simulink model "UAV_Dynamics"  (R2023b)
settings: Solver=ode4  StartTime=0.0  StopTime=inf  RelTol=1e-3
model workspace (MAT data in the model file):
  Horizontal_position_accuracy = 0.01
  Horizontal_position_accuracy_fault = Simulink.Parameter
  Horizontal_position_accuracy_fault.Value = 0
  Horizontal_position_accuracy_fault.DataType = 'auto'
  Horizontal_position_accuracy_fault.Complexity = 'real'
  Horizontal_position_accuracy_fault.Dimensions = [1 1]
  Velocity_accuracy = 0.01
  Velocity_accuracy_fault = Simulink.Parameter
  Velocity_accuracy_fault.Value = 0
  Velocity_accuracy_fault.DataType = 'auto'
  Velocity_accuracy_fault.Complexity = 'real'
  Velocity_accuracy_fault.Dimensions = [1 1]
  Vertical_position_accuracy = 0.01
  Vertical_position_accuracy_fault = Simulink.Parameter
  Vertical_position_accuracy_fault.Value = 0
  Vertical_position_accuracy_fault.DataType = 'auto'
  Vertical_position_accuracy_fault.Complexity = 'real'
  Vertical_position_accuracy_fault.Dimensions = [1 1]
  bias_acc = [0 0 0]
  bias_gyro = [0 0 0]
  mag_bias = [0 0 0]
undefined symbols (not defined in the file): contact, control, ddx, ddy, ddz, dragCoeffMov, dx, dy, dz, fractalcoef, g, m_to_mm, mass, p, pitch, q, r, ref_height, ref_lat, ref_lon, roll, rotorDir, rotorPositions, rotorThrustMax, rotorTimeConst, rotorTorqueMax, SampleTime, windVel, X, Y, yaw, Z
libraries: aerolibatmos2 x1, sensorgpslib x1, robotcorelib x1, mspsensorlib x1, shared6dof x1, simulink x1
(part 1 of 2)
settings Model: Creator=The MathWorks, Inc.  LastModifiedBy=cardo
settings SolverCC: ZeroCrossControl=EnableAll  MaxZcPerStep=1
settings OptimizationCC: ReuseModelBlockBuffer=off
settings ModelReferenceCC: EnableRefExpFcnMdlSchedulingChecks=on
settings RTWCC: DLArmComputeVersion=19.05

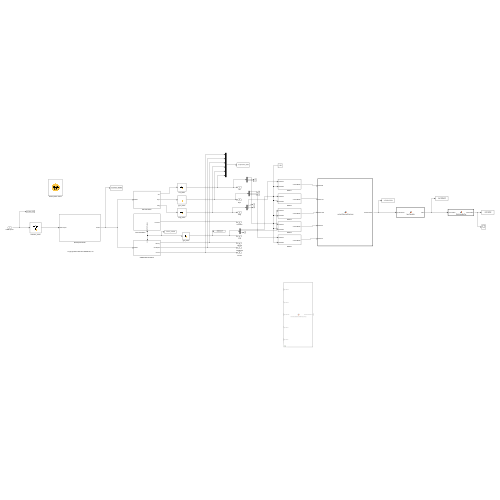
[thumbnail: Simulink's stored preview of the top-level diagram]
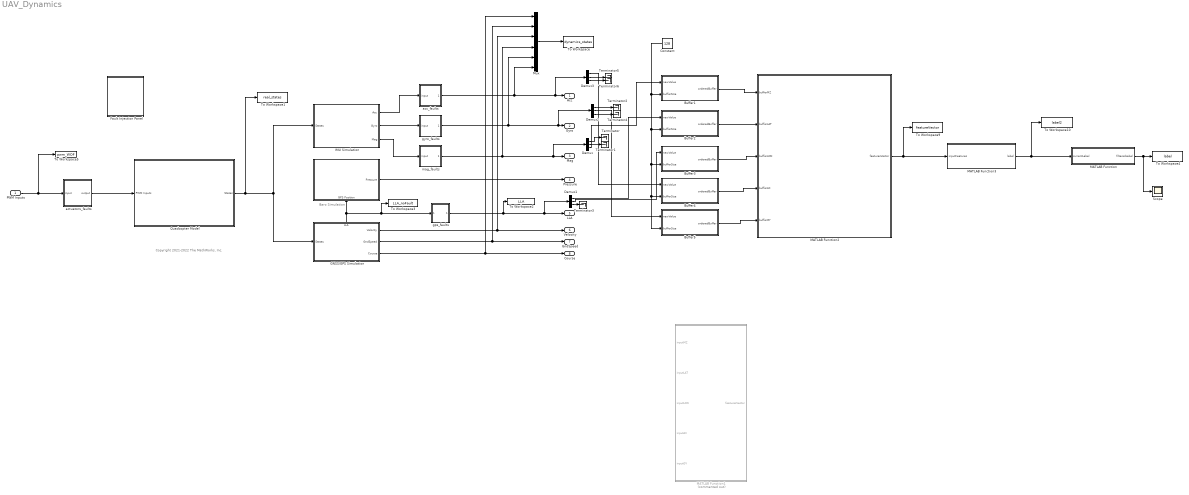
== system UAV_Dynamics ==
  note: Baro Simulation
  note: Copyright 2021-2022 The MathWorks, Inc.
  PWM Inputs : Inport
  " " : Subsystem
      settings: PortSchema="{\"entries\":[{\"content\":{\"sides\":[{\"content\":{\"connectorIds\":[]},\"type\":\"ConnectorPlacement.EquallySpacedRectSide\",\"uuid\":\"7ecc8b21-8f8f-4144-826a-6b68e30dbf7d\"},{\"content\":{\"connectorIds\":[\"Out1\"],\"side\":\"RIGHT\"},\"type\":\"ConnectorPlacement.EquallySpacedRectSide\",\"uuid\":\"81a1dd55-8330-4386-9921-36c0eb60d526\"},{\"content\":{\"connectorIds\":[],\"side\":\"TOP\"},\"type\":\"ConnectorPlacement.EquallySpacedRectSide\",\"uuid\":\"b99caff5-b40d-407d-b30e-35210c1aee1d\"},{\"content\":{\"connectorIds\":[\"In1\"],\"side\":\"BOTTOM\"},\"type\":\"ConnectorPlacement.EquallySpacedRectSide\",\"uuid\":\"18bfda3d-4fab-4e61-9ebc-e384e51de306\"}]},\"type\":\"ConnectorPlacement.EquallySpacedConnector\",\"uuid\":\"17ab4e96-b761-4c62-a0bb-ab626dac3eaa\"}],\"packageUris\":[\"http://schema.mathworks.com/mf0/Connector/R2020b\"],\"version\":\"1.0\"}"
  Buffer1 : Subsystem
  Buffer2 : Subsystem
  Buffer3 : Subsystem
  Buffer4 : Subsystem
  Buffer5 : Subsystem
  Constant : Constant  Value=128  SampleTime=0.01
  Demux{,1..3} (4 alike) : Demux  Outputs=3
  Fault Injection Panel : Subsystem
      mask DialogControl Container3 Prompt: Fault Injection
      mask DialogControl Control3 Prompt: Fault Injection Actuators
      mask DialogControl Control4 Prompt: Faut Injection Actuators
      mask DialogControl Control4 Callback: open_system('UAV_Dynamics/actuators_faults', 'mask');
      mask DialogControl Control5 Prompt: Fault Injection Sensors
      mask DialogControl Control6 Prompt: Fault Injection Accelometer
      mask DialogControl Control6 Callback: open_system('UAV_Dynamics/acc_faults', 'mask');
      mask DialogControl Control7 Prompt: Fault Injection Gyroscope
      mask DialogControl Control7 Callback: open_system('UAV_Dynamics/gyro_faults', 'mask');
      mask DialogControl Control8 Prompt: Fault Injection Magnometer
      mask DialogControl Control8 Callback: open_system('UAV_Dynamics/mag_faults', 'mask');
      mask DialogControl Control9 Prompt: Fault Injection GPS
      mask DialogControl Control9 Callback: open_system('UAV_Dynamics/gps_faults', 'mask');
  GNSS/GPS Simulation : Subsystem
      settings: PortSchema="{\"entries\":[{\"content\":{\"sides\":[{\"content\":{\"connectorIds\":[\"In1\"]},\"type\":\"ConnectorPlacement.EquallySpacedRectSide\",\"uuid\":\"4934e8ff-5d4b-4e11-968d-c23bd62383a0\"},{\"content\":{\"connectorIds\":[\"Out1\",\"Out2\",\"Out3\"],\"side\":\"RIGHT\"},\"type\":\"ConnectorPlacement.EquallySpacedRectSide\",\"uuid\":\"9ec8bc0a-2d3c-4dca-835c-010ac29b6ebc\"},{\"content\":{\"connectorIds\":[\"Out4\"],\"side\":\"TOP\"},\"type\":\"ConnectorPlacement.EquallySpacedRectSide\",\"uuid\":\"04f09eb4-1bd9-450e-b951-47054bdd92ad\"}]},\"type\":\"ConnectorPlacement.EquallySpacedConnector\",\"uuid\":\"9a5920cf-a58d-4c98-839b-fbac94edbe7e\"}],\"packageUris\":[\"http://schema.mathworks.com/mf0/Connector/R2020b\"],\"version\":\"1.0\"}"
  IMU Simulation : Subsystem
  MATLAB Function : MATLAB Function  TreatAsAtomicUnit=on
  MATLAB Function1 : MATLAB Function  Commented=on  TreatAsAtomicUnit=on
  MATLAB Function2 : MATLAB Function  TreatAsAtomicUnit=on
  MATLAB Function3 : MATLAB Function  TreatAsAtomicUnit=on
  Mux : Mux  Inputs=6
  Quadcopter Model : Subsystem
  Scope : Scope
  Terminator{,1..6} (7 alike) : Terminator
  To Workspace : ToWorkspace  VariableName=dynamics_states  SaveFormat=Timeseries  SampleTime=0.01
  To Workspace1 : ToWorkspace  VariableName=real_states  SaveFormat=Timeseries  SampleTime=0.01
  To Workspace10 : ToWorkspace  VariableName=label2  SaveFormat=Timeseries  SampleTime=-1
  To Workspace2 : ToWorkspace  VariableName=LLA  SaveFormat=Timeseries  SampleTime=0.01
  To Workspace3 : ToWorkspace  VariableName=LLA_noFault  SaveFormat=Timeseries  SampleTime=0.01
  To Workspace4 : ToWorkspace  VariableName=label  SaveFormat=Timeseries  SampleTime=-1
  To Workspace5 : ToWorkspace  VariableName=pwm_WOF  SaveFormat=Timeseries  SampleTime=0.01
  To Workspace9 : ToWorkspace  VariableName=featureVector  SaveFormat=Timeseries  SampleTime=-1
  acc_faults : Subsystem  mask{tf=100, freezingX=off, freezingY=off, freezingZ=off, accuracyX=off, accuracyY=off, accuracyZ=off, d_accuracy=10.0, driftX=off, driftY=off, driftZ=off, landa=0.07, biasX=off, bias_ax=0, biasY=off, bias_ay=0.01, biasZ=off, bias_az=0}
      mask prompts: tf "Fault Time(s):"; freezingX "Freezing Fault ax On"; freezingY "Freezing Fault ay On"; freezingZ "Freezing Fault az On"; accuracyX "Accuracy Fault ax On"; accuracyY "Accuracy Fault ay On"; accuracyZ "Accuracy Fault az On"; d_accuracy "Accuracy Error max, dmax (%):"; driftX "Drift Fault ax On"; driftY "Drift Fault ay On"; driftZ "Drift Fault az On"; landa "Lambda:"; biasX "Bias Fault ax On"; bias_ax "Bias Offset ax (m/s²):"; biasY "Bias Fault ay On"; bias_ay "Bias Offset ay (m/s²):"; biasZ "Bias Fault az On"; bias_az "Bias Offset az (m/s²):"
      mask TypeOptions tf: tf/Value
      mask DialogControl Control5 Prompt: Fault Injection Accelerometer
      mask DialogControl Container7 Prompt: Fault Time
      mask DialogControl Control4 Prompt: Insert the Fault Time
      mask DialogControl ParameterGroupVar Prompt: Fault Type
      mask DialogControl DescTextVar Prompt: Select the type of Fault,its amplitude and the relative axis
      mask DialogControl Container4 Prompt: Freezing Fault
      mask DialogControl Control6_copy_copy Prompt: Insert Freezing Fault
      mask DialogControl Container5 Prompt: Accuracy Fault
      mask DialogControl Control6_copy_copy_copy Prompt: Insert Accuracy Fault. Select the axis with the Fault and write the percent of max error
      mask DialogControl Control3 Prompt: y(t) = x(t) + d(t), |d(t)| ≤ dmax, for all t ≥ tf
      mask DialogControl Container6 Prompt: Drift Fault
      mask DialogControl Control6_copy Prompt: Insert Drift Offset Fault. Select the axis with the Fault and write the value of lambda.
      mask DialogControl Control2 Prompt: y(t) = x(t) + d(t), |d(t)| = λ*t, 0 < λ << 1, for all t ≥ tf
      mask DialogControl Container8 Prompt: Bias Fault
      mask DialogControl Control6 Prompt: Insert Bias Offset Fault
      mask Display: image('accelometer_fault_icon.png');
  actuators_faults : Subsystem  mask{tf=150, num_motor=No Fault, lock_in_place=off, float=off, handover=off, loss_effectiveness=off, perc=30}
      mask prompts: tf "Fault Time(s):"; lock_in_place "Lock in Place Fault On"; float "Float Fault On"; handover "Handover Fault On"; loss_effectiveness "Loss of Effectiveness Fault On"; perc "Percentage of Fault (%):"
      mask TypeOptions tf: tf/Value
      mask DialogControl DescTextVar Prompt: Actuators Fault Injection
      mask DialogControl ParameterGroupVar Prompt: Fault Time and Motor
      mask DialogControl Control2 Prompt: Insert the fault time
      mask DialogControl Control3 Prompt: Insert the actuator with the fault
      mask DialogControl Container3 Prompt: Fault Type
      mask DialogControl Container5 Prompt: Lock in Place
      mask DialogControl Container6 Prompt: Float
      mask DialogControl Container7 Prompt: Handover
      mask DialogControl Container8 Prompt: Loss of Effectiveness
      mask Display: image('motor_fault.png');
  gps_faults : Subsystem  mask{tf=100, loss_signal=off, lossProbability=20, gps_accuracy=on, AccuracyErrorMeters=5}
      mask prompts: tf "Fault Time (s):"; loss_signal "Packet Loss Signal On"; lossProbability "Probability of Packet Loss of Signal"; gps_accuracy "GPS Fault On"; AccuracyErrorMeters "Error Position accuracy (m):"
      mask TypeOptions tf: tf/Value
      mask DialogControl Control5 Prompt: Fault Injection GPS
      mask DialogControl Container7 Prompt: Fault Time
      mask DialogControl Control4 Prompt: Insert the fault time
      mask DialogControl ParameterGroupVar Prompt: Fault
      mask DialogControl DescTextVar Prompt: Select the Fault Type and its amplitude
      mask DialogControl Container8 Prompt: Packet Loss of Signal
      mask DialogControl Container5 Prompt: GPS Accuracy
      mask Display: image('gps_fault_icon.png');
  gyro_faults : Subsystem  mask{tf=100, freezingX=off, freezingY=off, freezingZ=off, accuracyX=off, accuracyY=off, accuracyZ=off, d_accuracy=10.0, driftX=off, driftY=off, driftZ=off, landa=0.01, biasX=off, bias_gx=0, biasY=off, bias_gy=0.06, biasZ=off, bias_gz=0}
      mask prompts: tf "Fault Time (s):"; freezingX "Freezing Fault gx On"; freezingY "Freezing Fault gy On"; freezingZ "Freezing Fault gz On"; accuracyX "Accuracy Fault gx On"; accuracyY "Accuracy Fault gy On"; accuracyZ "Accuracy Fault gz On"; d_accuracy "Accuracy Error max, dmax (%):"; driftX "Drift Fault gx On"; driftY "Drift Fault gy On"; driftZ "Drift Fault gz On"; landa "Lambda"; biasX "Bias Fault gx On"; bias_gx "Bias Offset gx (rad/s):"; biasY "Bias Fault gy On"; bias_gy "Bias Offset gy (rad/s):"; biasZ "Bias Fault gz On"; bias_gz "Bias Offset gz (rad/s):"
      mask TypeOptions tf: tf/Value
      mask DialogControl Control5 Prompt: Fault Injection Gyroscope
      mask DialogControl Container7 Prompt: Fault Time
      mask DialogControl Control4 Prompt: Insert the Fault Time
      mask DialogControl ParameterGroupVar Prompt: Fault Type
      mask DialogControl DescTextVar Prompt: Select the type of Fault,its amplitude and the relative axis
      mask DialogControl Container4 Prompt: Freezing Fault
      mask DialogControl Control6_copy_copy Prompt: Insert Freezing Fault
      mask DialogControl Container5 Prompt: Accuracy Fault
      mask DialogControl Control6_copy_copy_copy Prompt: Insert Accuracy Fault. Select the axis with the Fault and write the percent of max error
      mask DialogControl Control3 Prompt: y(t) = x(t) + d(t), |d(t)| ≤ dmax, for all t ≥ tf
      mask DialogControl Container6 Prompt: Drift Fault
      mask DialogControl Control6_copy Prompt: Insert Drift Offset Fault. Select the axis with the Fault and write the value of lambda.
      mask DialogControl Control2 Prompt: y(t) = x(t) + d(t), |d(t)| = λ*t, 0 < λ << 1, for all t ≥ tf
      mask DialogControl Container8 Prompt: Bias Fault
      mask DialogControl Control6 Prompt: Insert Bias Offset Fault
      mask Display: image('gyroscope_fault_icon.png');
  mag_faults : Subsystem  mask{tf=100, freezingX=off, freezingY=off, freezingZ=off, accuracyX=off, accuracyY=off, accuracyZ=off, d_accuracy=20, driftX=off, driftY=off, driftZ=off, landa=0.1, biasX=off, bias_mx=0, biasY=off, bias_my=0, biasZ=off, bias_mz=0}
      mask prompts: tf "Fault Time (s):"; freezingX "Freezing Fault mx On"; freezingY "Freezing Fault my On"; freezingZ "Freezing Fault mz On"; accuracyX "Accuracy Fault mx On"; accuracyY "Accuracy Fault my On"; accuracyZ "Accuracy Fault mz On"; d_accuracy "Accuracy Error max, dmax (%):"; driftX "Drift Fault mx On"; driftY "Drift Fault my On"; driftZ "Drift Fault mz On"; landa "Lambda:"; biasX "Bias Fault mx On"; bias_mx "Bias Offset mx (µT):"; biasY "Bias Fault my On"; bias_my "Bias Offset my (µT):"; biasZ "Bias Fault mz On"; bias_mz "Bias Offset mz (µT):"
      mask TypeOptions tf: tf/Value
      mask DialogControl Control5 Prompt: Fault Injection Magnometer
      mask DialogControl Container7 Prompt: Fault Time
      mask DialogControl Control4 Prompt: Insert the Fault Time
      mask DialogControl ParameterGroupVar Prompt: Fault Type
      mask DialogControl DescTextVar Prompt: Select the type of Fault,its amplitude and the relative axis
      mask DialogControl Container4 Prompt: Freezing Fault
      mask DialogControl Control6_copy_copy Prompt: Insert Freezing Fault
      mask DialogControl Container5 Prompt: Accuracy Fault
      mask DialogControl Control6_copy_copy_copy Prompt: Insert Accuracy Fault. Select the axis with the Fault and write the percent of max error
      mask DialogControl Control3 Prompt: y(t) = x(t) + d(t), |d(t)| ≤ dmax, for all t ≥ tf
      mask DialogControl Container6 Prompt: Drift Fault
      mask DialogControl Control6_copy Prompt: Insert Drift Offset Fault. Select the axis with the Fault and write the value of lambda.
      mask DialogControl Control2 Prompt: y(t) = x(t) + d(t), |d(t)| = λ*t, 0 < λ << 1, for all t ≥ tf
      mask DialogControl Container8 Prompt: Bias Fault
      mask DialogControl Control6 Prompt: Insert Bias Offset Fault
      mask Display: image('magnometer_fault_icon.png');
  Acc : Outport
  Gyro : Outport  Port=2
  Mag : Outport  Port=3
  Pressure : Outport  Port=4
  LLA : Outport  Port=5
  Velocity : Outport  Port=6
  GndSpeed : Outport  Port=7
  Course : Outport  Port=8
  wires:
  IMU Simulation/2(Gyro) -> gyro_faults/1(input)
  IMU Simulation/3(Mag) -> mag_faults/1(input)
  " "/1(Pressure) -> Pressure/1
  GNSS/GPS Simulation/1(Velocity) -> Mux/3, Velocity/1
  GNSS/GPS Simulation/2(GndSpeed) -> Mux/2, GndSpeed/1
  GNSS/GPS Simulation/3(Course) -> Mux/1, Course/1
  Mux/1 -> To Workspace/1
  IMU Simulation/1(Acc) -> acc_faults/1(input)
  actuators_faults/1(output) -> Quadcopter Model/1(PWM Inputs)
  mag_faults/1(output) -> Mux/4, Demux/1, Mag/1
  GNSS/GPS Simulation/4(LLA) -> gps_faults/1(input), To Workspace3/1, " "/1(GPS Position)
  Quadcopter Model/1(States) -> To Workspace1/1, GNSS/GPS Simulation/1(States), IMU Simulation/1(States)
  Demux/1 -> Terminator/1
  Demux/2 -> Terminator1/1
  PWM Inputs/1 -> To Workspace5/1, actuators_faults/1(input)
  Demux2/3 -> Terminator4/1
  gyro_faults/1(output) -> Mux/5, Demux2/1, Gyro/1
  Demux2/1 -> Terminator2/1
  acc_faults/1(output) -> Mux/6, Demux3/1, Acc/1
  Demux3/3 -> Terminator6/1
  gps_faults/1(output) -> Demux1/1, LLA/1, To Workspace2/1
  Demux1/3 -> Terminator3/1
  Demux3/2 -> Terminator5/1
  MATLAB Function3/1(label) -> MATLAB Function/1(currentLabel), To Workspace10/1
  Buffer4/1(orderedBuffer) -> MATLAB Function2/4(bufferAX)
  Buffer5/1(orderedBuffer) -> MATLAB Function2/5(bufferGY)
  Buffer3/1(orderedBuffer) -> MATLAB Function2/3(bufferLON)
  Buffer1/1(orderedBuffer) -> MATLAB Function2/1(bufferMZ)
  Buffer2/1(orderedBuffer) -> MATLAB Function2/2(bufferLAT)
  Constant/1 -> Buffer1/2(bufferSize), Buffer2/2(bufferSize), Buffer3/2(bufferSize), Buffer4/2(bufferSize), Buffer5/2(bufferSize)
  Demux/3 -> Buffer1/1(newValue)
  Demux1/1 -> Buffer2/1(newValue)
  Demux1/2 -> Buffer3/1(newValue)
  Demux3/1 -> Buffer4/1(newValue)
  Demux2/2 -> Buffer5/1(newValue)
  MATLAB Function2/1(featuresVector) -> MATLAB Function3/1(inputFeatures), To Workspace9/1
  MATLAB Function/1(filteredLabel) -> Scope/1, To Workspace4/1

== system UAV_Dynamics/  ==
  GPS Position : Inport
  Extract Altitude : Selector  InputPortWidth=3  IndexOptions=Index vector (dialog)  Indices=[3]  OutputSizes=1
  Gain1 : Gain  Gain=1/m_to_mm
  Gain2 : Gain  Gain=m_to_mm
  Lapse Rate Model : aerolibatmos2/ISA Atmosphere Model  useExtended=off  action=Warning  custom=on  viscosityOut=off  g=9.80665  gamma=1.4  R=287.0531  L=0.0065  h_trop=11000  h_strat=20000  rho0=1.225  P0=101325  T0=288.15  h0=0
  Random Number1 : RandomNumber  Variance=10000  Seed=10  SampleTime=SampleTime
  Sum1 : Sum  Inputs=|++
  Terminator : Terminator
  Terminator1 : Terminator
  Terminator2 : Terminator
  Pressure : Outport
  wires:
  Lapse Rate Model/2 -> Terminator1/1
  Lapse Rate Model/4 -> Terminator2/1
  Lapse Rate Model/1 -> Terminator/1
  Lapse Rate Model/3 -> Pressure/1
  Sum1/1 -> Gain1/1
  Gain2/1 -> Sum1/1
  Extract Altitude/1 -> Gain2/1
  Gain1/1 -> Lapse Rate Model/1
  GPS Position/1 -> Extract Altitude/1
  Random Number1/1 -> Sum1/2  "Pressure_noise"

== system UAV_Dynamics/Buffer1 ==
  newValue : Inport
  bufferSize : Inport  Port=2
  Delay : Delay  DelayLength=1  InitialCondition=1
  Delay1 : Delay  DelayLength=1  InitialCondition=zeros(128,1)
  MATLAB Function : MATLAB Function  TreatAsAtomicUnit=on
  MATLAB Function2 : MATLAB Function  TreatAsAtomicUnit=on
  orderedBuffer : Outport
  wires:
  newValue/1 -> MATLAB Function/2(newValue)
  MATLAB Function/1(buffer) -> Delay1/1, MATLAB Function2/1(buffer)
  MATLAB Function2/1(orderedBuffer) -> orderedBuffer/1
  MATLAB Function/2(k) -> Delay/1, MATLAB Function2/2(k)
  Delay/1 -> MATLAB Function/4("k ")
  Delay1/1 -> MATLAB Function/1("buffer ")
  bufferSize/1 -> MATLAB Function/3(bufferSize)

== system UAV_Dynamics/Buffer2 ==
  newValue : Inport
  bufferSize : Inport  Port=2
  Delay : Delay  DelayLength=1  InitialCondition=1
  Delay1 : Delay  DelayLength=1  InitialCondition=zeros(128,1)
  MATLAB Function : MATLAB Function  TreatAsAtomicUnit=on
  MATLAB Function2 : MATLAB Function  TreatAsAtomicUnit=on
  orderedBuffer : Outport
  wires:
  newValue/1 -> MATLAB Function/2(newValue)
  MATLAB Function/1(buffer) -> Delay1/1, MATLAB Function2/1(buffer)
  MATLAB Function2/1(orderedBuffer) -> orderedBuffer/1
  MATLAB Function/2(k) -> Delay/1, MATLAB Function2/2(k)
  Delay/1 -> MATLAB Function/4("k ")
  Delay1/1 -> MATLAB Function/1("buffer ")
  bufferSize/1 -> MATLAB Function/3(bufferSize)

== system UAV_Dynamics/Buffer3 ==
  newValue : Inport
  bufferSize : Inport  Port=2
  Delay : Delay  DelayLength=1  InitialCondition=1
  Delay1 : Delay  DelayLength=1  InitialCondition=zeros(128,1)
  MATLAB Function : MATLAB Function  TreatAsAtomicUnit=on
  MATLAB Function2 : MATLAB Function  TreatAsAtomicUnit=on
  orderedBuffer : Outport
  wires:
  newValue/1 -> MATLAB Function/2(newValue)
  MATLAB Function/1(buffer) -> Delay1/1, MATLAB Function2/1(buffer)
  MATLAB Function2/1(orderedBuffer) -> orderedBuffer/1
  MATLAB Function/2(k) -> Delay/1, MATLAB Function2/2(k)
  Delay/1 -> MATLAB Function/4("k ")
  Delay1/1 -> MATLAB Function/1("buffer ")
  bufferSize/1 -> MATLAB Function/3(bufferSize)

== system UAV_Dynamics/Buffer4 ==
  newValue : Inport
  bufferSize : Inport  Port=2
  Delay : Delay  DelayLength=1  InitialCondition=1
  Delay1 : Delay  DelayLength=1  InitialCondition=zeros(128,1)
  MATLAB Function : MATLAB Function  TreatAsAtomicUnit=on
  MATLAB Function2 : MATLAB Function  TreatAsAtomicUnit=on
  orderedBuffer : Outport
  wires:
  newValue/1 -> MATLAB Function/2(newValue)
  MATLAB Function/1(buffer) -> Delay1/1, MATLAB Function2/1(buffer)
  MATLAB Function2/1(orderedBuffer) -> orderedBuffer/1
  MATLAB Function/2(k) -> Delay/1, MATLAB Function2/2(k)
  Delay/1 -> MATLAB Function/4("k ")
  Delay1/1 -> MATLAB Function/1("buffer ")
  bufferSize/1 -> MATLAB Function/3(bufferSize)

== system UAV_Dynamics/Buffer5 ==
  newValue : Inport
  bufferSize : Inport  Port=2
  Delay : Delay  DelayLength=1  InitialCondition=1
  Delay1 : Delay  DelayLength=1  InitialCondition=zeros(128,1)
  MATLAB Function : MATLAB Function  TreatAsAtomicUnit=on
  MATLAB Function2 : MATLAB Function  TreatAsAtomicUnit=on
  orderedBuffer : Outport
  wires:
  newValue/1 -> MATLAB Function/2(newValue)
  MATLAB Function/1(buffer) -> Delay1/1, MATLAB Function2/1(buffer)
  MATLAB Function2/1(orderedBuffer) -> orderedBuffer/1
  MATLAB Function/2(k) -> Delay/1, MATLAB Function2/2(k)
  Delay/1 -> MATLAB Function/4("k ")
  Delay1/1 -> MATLAB Function/1("buffer ")
  bufferSize/1 -> MATLAB Function/3(bufferSize)

== system UAV_Dynamics/Fault Injection Panel ==

== system UAV_Dynamics/GNSS//GPS Simulation ==
  States : Inport
  Bus Selector : BusSelector  OutputSignals=dx,dy,dz  OutputAsBus=on
  Bus Selector1 : BusSelector  OutputSignals=X,Y,Z  OutputAsBus=on
  GPS : sensorgpslib/GPS  DispRefFrame=NED  PositionInputFormat=Local  ReferenceLocation=[ref_lat ref_lon ref_height]  HorizontalPositionAccuracy=0.01  VerticalPositionAccuracy=0.01  VelocityAccuracy=0.01  DecayFactor=0.99  SeedDouble=67  SimulateUsing=Code generation
  Reshape1 : Reshape  OutputDimensionality=Row vector (2-D)
  Reshape3 : Reshape  OutputDimensionality=Row vector (2-D)
  Velocity : Outport
  GndSpeed : Outport  Port=2
  Course : Outport  Port=3
  LLA : Outport  Port=4
  wires:
  Reshape3/1 -> GPS/1
  GPS/1 -> LLA/1  "lla"
  Bus Selector1/1 -> Reshape3/1
  Bus Selector/1 -> Reshape1/1
  Reshape1/1 -> GPS/2
  GPS/2 -> Velocity/1
  States/1 -> Bus Selector/1, Bus Selector1/1
  GPS/3 -> GndSpeed/1
  GPS/4 -> Course/1

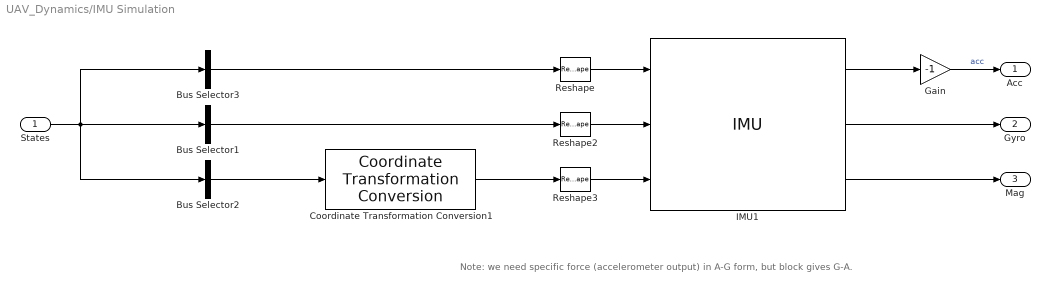
== system UAV_Dynamics/IMU Simulation ==
  note: Note:
      | we need specific force (accelerometer output) in A-G form, but block gives G-A.
  States : Inport
  Bus Selector1 : BusSelector  OutputSignals=p,q,r  OutputAsBus=on
  Bus Selector2 : BusSelector  OutputSignals=yaw,pitch,roll  OutputAsBus=on
  Bus Selector3 : BusSelector  OutputSignals=ddx,ddy,ddz  OutputAsBus=on
  Coordinate Transformation Conversion1 : robotcorelib/Coordinate Transformation Conversion  InputRepresentation=Euler Angles  InputEulerSequence=ZYX  ShowTrVecInputPort=on  OutputRepresentation=Quaternion  OutputEulerSequence=ZYX  ShowTrVecOutputPort=on  SimulateUsing=Interpreted execution
  Gain : Gain  Gain=-1
  IMU1 : mspsensorlib/IMU  DispRefFrame=NED  TemperaturePort=off  Temperature=25  MagneticFieldPort=off  MagneticFieldNED=[21.5 1.16 43.1]  MagneticFieldENU=[ -2.4169, 27.5550, 16.0849 ]  SeedDouble=87254  SimulateUsing=Interpreted execution  AccelParamsMeasurementRange=Inf  AccelParamsResolution=0  AccelParamsConstantBias=[ 0, 0, 0]  AccelParamsAxesMisalignment=[ 0, 0, 0 ]  AccelParamsNoiseDensity=0.0003  AccelParamsBiasInstability=[ 0, 0, 0 ]  AccelParamsBiasInstabilityNumerator=fractalcoef().Numerator  AccelParamsBiasInstabilityDenominator=fractalcoef().Denominator  AccelParamsRandomWalk=[ 0, 0, 0 ]  AccelParamsNoiseType=double-sided  AccelParamsTemperatureBias=[ 0, 0, 0 ]  AccelParamsTemperatureScaleFactor=[ 0, 0, 0 ]  GyroParamsMeasurementRange=Inf  GyroParamsResolution=0  GyroParamsConstantBias=[ 0, 0, 0]  GyroParamsAxesMisalignment=[ 0, 0, 0 ]  GyroParamsAccelerationBias=0.0001  GyroParamsNoiseDensity=0.01  GyroParamsBiasInstability=[ 0, 0, 0 ]  GyroParamsBiasInstabilityNumerator=fractalcoef().Numerator  GyroParamsBiasInstabilityDenominator=fractalcoef().Denominator  GyroParamsRandomWalk=[ 0, 0, 0 ]  GyroParamsNoiseType=double-sided  GyroParamsTemperatureBias=[ 0, 0, 0 ]  GyroParamsTemperatureScaleFactor=[ 0, 0, 0 ]  MagParamsMeasurementRange=Inf  MagParamsResolution=0  MagParamsConstantBias=[ 0, 0, 0]  MagParamsAxesMisalignment=[ 0, 0, 0 ]  MagParamsNoiseDensity=0.0005  MagParamsBiasInstability=[ 0, 0, 0 ]  MagParamsBiasInstabilityNumerator=fractalcoef().Numerator  MagParamsBiasInstabilityDenominator=fractalcoef().Denominator  MagParamsRandomWalk=[ 0, 0, 0 ]  MagParamsNoiseType=double-sided  MagParamsTemperatureBias=[ 0, 0, 0 ]  MagParamsTemperatureScaleFactor=[ 0, 0, 0 ]
  Reshape : Reshape  OutputDimensionality=Row vector (2-D)
  Reshape2 : Reshape  OutputDimensionality=Row vector (2-D)
  Reshape3 : Reshape  OutputDimensionality=Row vector (2-D)
  Acc : Outport
  Gyro : Outport  Port=2
  Mag : Outport  Port=3
  wires:
  Coordinate Transformation Conversion1/1 -> Reshape3/1
  Reshape3/1 -> IMU1/3
  IMU1/3 -> Mag/1
  IMU1/2 -> Gyro/1
  Reshape/1 -> IMU1/1
  Bus Selector3/1 -> Reshape/1
  IMU1/1 -> Gain/1
  Bus Selector1/1 -> Reshape2/1
  Bus Selector2/1 -> Coordinate Transformation Conversion1/1
  Reshape2/1 -> IMU1/2
  States/1 -> Bus Selector1/1, Bus Selector2/1, Bus Selector3/1
  Gain/1 -> Acc/1  "acc"

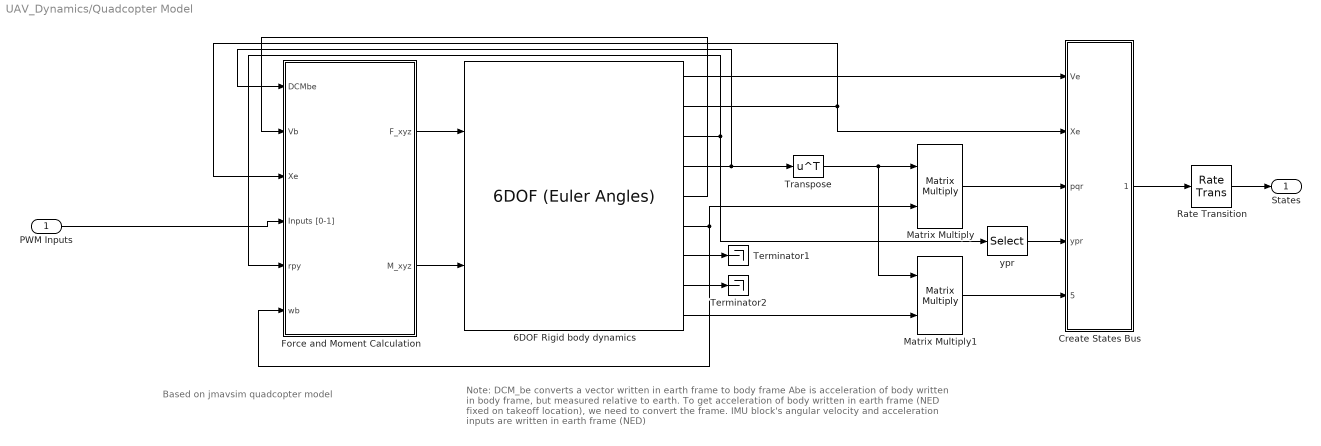
== system UAV_Dynamics/Quadcopter Model ==
  note: Note:
      | DCM_be converts a vector written in earth frame to body frame
      | Abe is acceleration of body written in body frame, but measured relative to earth.
      | To get acceleration of body written in earth frame (NED fixed on takeoff location), we need to convert the frame.
      | IMU block's angular velocity and acceleration inputs are written in earth frame (NED)
  note: Based on jmavsim quadcopter model
  PWM Inputs : Inport
  "6DOF Rigid body dynamics " : shared6dof/6DOF (Euler Angles)  units=Metric (MKS)  mtype=Fixed  rep=Quaternion  xme_0=init.posNED  Vm_0=init.vb  eul_0=init.euler  pm_0=init.angRates  mass_0=mass  mass_e=0.5  mass_f=2.0  inertia=inertia  inertia_e=eye(3)  inertia_f=2*eye(3)  k_quat=1  vre_flag=on  abi_flag=on  aMode=aMode  xme_statename=''  Vm_statename=''  eul_statename=''  quat_statename=''  pm_statename=''  mass_statename=''
  Create States Bus : Subsystem
  Force and Moment Calculation : Subsystem
  Matrix Multiply : Product  Multiplication=Matrix(*)
  Matrix Multiply1 : Product  Multiplication=Matrix(*)
  Rate Transition : RateTransition  OutPortSampleTime=SampleTime
  Terminator1 : Terminator
  Terminator2 : Terminator
  Transpose : Math  Operator=transpose
  ypr : Selector  InputPortWidth=3  IndexOptions=Index vector (dialog)  Indices=[3 2 1]  OutputSizes=1
  States : Outport
  wires:
  Matrix Multiply/1 -> Create States Bus/3(pqr)
  "6DOF Rigid body dynamics "/6 -> Matrix Multiply/2, Force and Moment Calculation/6(wb)
  Force and Moment Calculation/1(F_xyz) -> "6DOF Rigid body dynamics "/1
  "6DOF Rigid body dynamics "/9 -> Matrix Multiply1/2
  Transpose/1 -> Matrix Multiply1/1, Matrix Multiply/1
  "6DOF Rigid body dynamics "/5 -> Force and Moment Calculation/2(Vb)
  ypr/1 -> Create States Bus/4(ypr)
  "6DOF Rigid body dynamics "/2 -> Force and Moment Calculation/3(Xe), Create States Bus/2(Xe)
  "6DOF Rigid body dynamics "/3 -> Force and Moment Calculation/5(rpy), ypr/1
  Rate Transition/1 -> States/1
  Create States Bus/1(States) -> Rate Transition/1
  "6DOF Rigid body dynamics "/7 -> Terminator1/1
  "6DOF Rigid body dynamics "/1 -> Create States Bus/1(Ve)
  "6DOF Rigid body dynamics "/8 -> Terminator2/1
  Force and Moment Calculation/2(M_xyz) -> "6DOF Rigid body dynamics "/2
  "6DOF Rigid body dynamics "/4 -> Force and Moment Calculation/1(DCMbe), Transpose/1
  Matrix Multiply1/1 -> Create States Bus/5(acc_lnav)
  PWM Inputs/1 -> Force and Moment Calculation/4(Inputs [0-1])

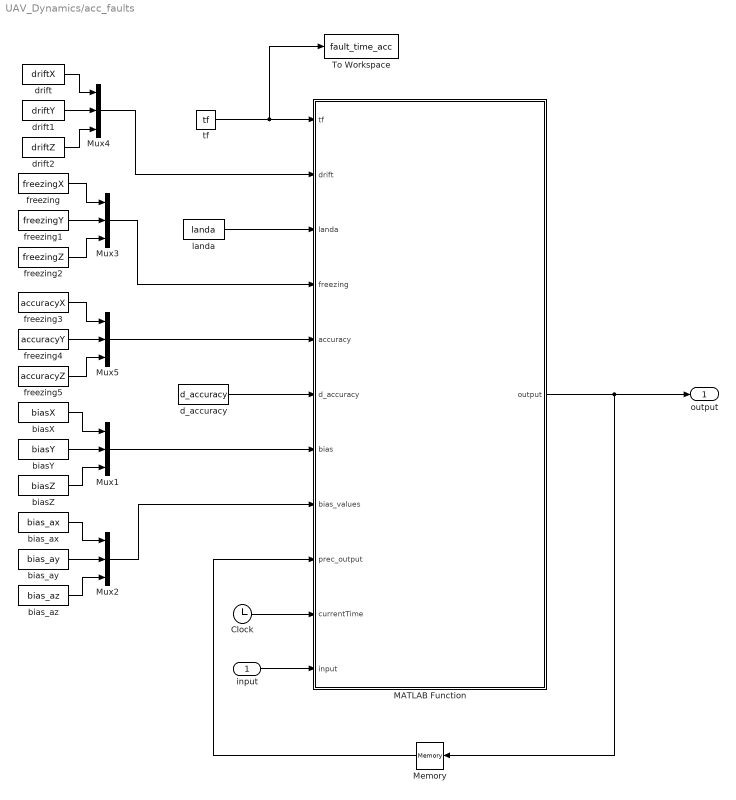
== system UAV_Dynamics/acc_faults ==
  input : Inport
  Clock : Clock
  MATLAB Function : MATLAB Function  TreatAsAtomicUnit=on
  Memory : Memory
  Mux{1..5} (5 alike) : Mux  Inputs=3
  To Workspace : ToWorkspace  VariableName=fault_time_acc  SaveFormat=Timeseries  SampleTime=0.01
  biasX : Constant  Value=biasX  SampleTime=0.01
  biasY : Constant  Value=biasY  SampleTime=0.01
  biasZ : Constant  Value=biasZ  SampleTime=0.01
  bias_ax : Constant  Value=bias_ax  SampleTime=0.01
  bias_ay : Constant  Value=bias_ay  SampleTime=0.01
  bias_az : Constant  Value=bias_az  SampleTime=0.01
  d_accuracy : Constant  Value=d_accuracy  SampleTime=0.01
  drift : Constant  Value=driftX  SampleTime=0.01
  drift1 : Constant  Value=driftY  SampleTime=0.01
  drift2 : Constant  Value=driftZ  SampleTime=0.01
  freezing : Constant  Value=freezingX  SampleTime=0.01
  freezing1 : Constant  Value=freezingY  SampleTime=0.01
  freezing2 : Constant  Value=freezingZ  SampleTime=0.01
  freezing3 : Constant  Value=accuracyX  SampleTime=0.01
  freezing4 : Constant  Value=accuracyY  SampleTime=0.01
  freezing5 : Constant  Value=accuracyZ  SampleTime=0.01
  landa : Constant  Value=landa  SampleTime=0.01
  tf : Constant  Value=tf
  output : Outport
  wires:
  input/1 -> MATLAB Function/11(input)
  MATLAB Function/1(output) -> output/1, Memory/1
  Memory/1 -> MATLAB Function/9(prec_output)
  d_accuracy/1 -> MATLAB Function/6(d_accuracy)
  Clock/1 -> MATLAB Function/10(currentTime)
  landa/1 -> MATLAB Function/3(landa)
  tf/1 -> MATLAB Function/1(tf), To Workspace/1
  biasX/1 -> Mux1/1
  biasY/1 -> Mux1/2
  biasZ/1 -> Mux1/3
  bias_ax/1 -> Mux2/1
  bias_ay/1 -> Mux2/2
  bias_az/1 -> Mux2/3
  Mux1/1 -> MATLAB Function/7(bias)
  Mux2/1 -> MATLAB Function/8(bias_values)
  freezing/1 -> Mux3/1
  freezing1/1 -> Mux3/2
  freezing2/1 -> Mux3/3
  Mux3/1 -> MATLAB Function/4(freezing)
  drift/1 -> Mux4/1
  drift1/1 -> Mux4/2
  drift2/1 -> Mux4/3
  Mux4/1 -> MATLAB Function/2(drift)
  freezing3/1 -> Mux5/1
  freezing4/1 -> Mux5/2
  freezing5/1 -> Mux5/3
  Mux5/1 -> MATLAB Function/5(accuracy)

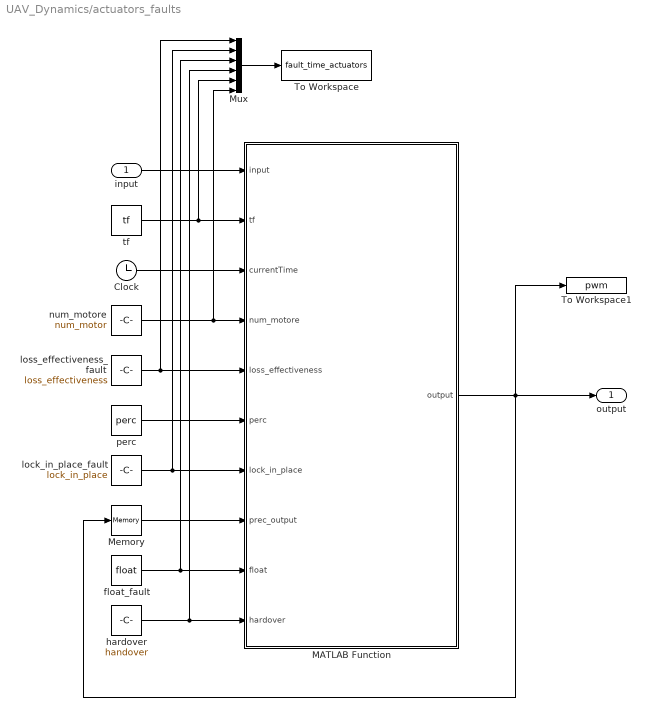
== system UAV_Dynamics/actuators_faults ==
  input : Inport
  Clock : Clock
  MATLAB Function : MATLAB Function  TreatAsAtomicUnit=on
  Memory : Memory
  Mux : Mux  Inputs=6
  To Workspace : ToWorkspace  VariableName=fault_time_actuators  SaveFormat=Timeseries  SampleTime=0.01
  To Workspace1 : ToWorkspace  VariableName=pwm  SaveFormat=Timeseries  SampleTime=0.01
  float_fault : Constant  Value=float
  hardover : Constant  Value=handover
  lock_in_place_fault : Constant  Value=lock_in_place
  loss_effectiveness_fault : Constant  Value=loss_effectiveness
  num_motore : Constant  Value=num_motor
  perc : Constant  Value=perc
  tf : Constant  Value=tf
  output : Outport
  wires:
  MATLAB Function/1(output) -> output/1, To Workspace1/1, Memory/1
  float_fault/1 -> MATLAB Function/9(float), Mux/3
  loss_effectiveness_fault/1 -> Mux/1, MATLAB Function/5(loss_effectiveness)
  hardover/1 -> MATLAB Function/10(hardover), Mux/4
  lock_in_place_fault/1 -> MATLAB Function/7(lock_in_place), Mux/2
  perc/1 -> MATLAB Function/6(perc)
  num_motore/1 -> MATLAB Function/4(num_motore), Mux/6
  input/1 -> MATLAB Function/1(input)
  Mux/1 -> To Workspace/1
  Memory/1 -> MATLAB Function/8(prec_output)
  tf/1 -> MATLAB Function/2(tf), Mux/5
  Clock/1 -> MATLAB Function/3(currentTime)

== system UAV_Dynamics/gps_faults ==
  input : Inport
  Clock : Clock
  HPA : Constant  Value=AccuracyErrorMeters  SampleTime=0.01
  MATLAB Function : MATLAB Function  TreatAsAtomicUnit=on
  To Workspace : ToWorkspace  VariableName=fault_time_gps  SaveFormat=Timeseries  SampleTime=0.01
  gps_accuracy : Constant  Value=gps_accuracy  SampleTime=0.01
  lossProbability : Constant  Value=lossProbability  SampleTime=0.01
  loss_signal : Constant  Value=loss_signal  SampleTime=0.01
  tf : Constant  Value=tf
  output : Outport
  wires:
  input/1 -> MATLAB Function/6(input)
  MATLAB Function/1(output) -> output/1
  loss_signal/1 -> MATLAB Function/3(loss_signal)
  Clock/1 -> MATLAB Function/5(currentTime)
  tf/1 -> MATLAB Function/1(tf), To Workspace/1
  lossProbability/1 -> MATLAB Function/4(lossProbability)
  gps_accuracy/1 -> MATLAB Function/2(gps_accuracy)
  HPA/1 -> MATLAB Function/7(accuracyErrorMeters)

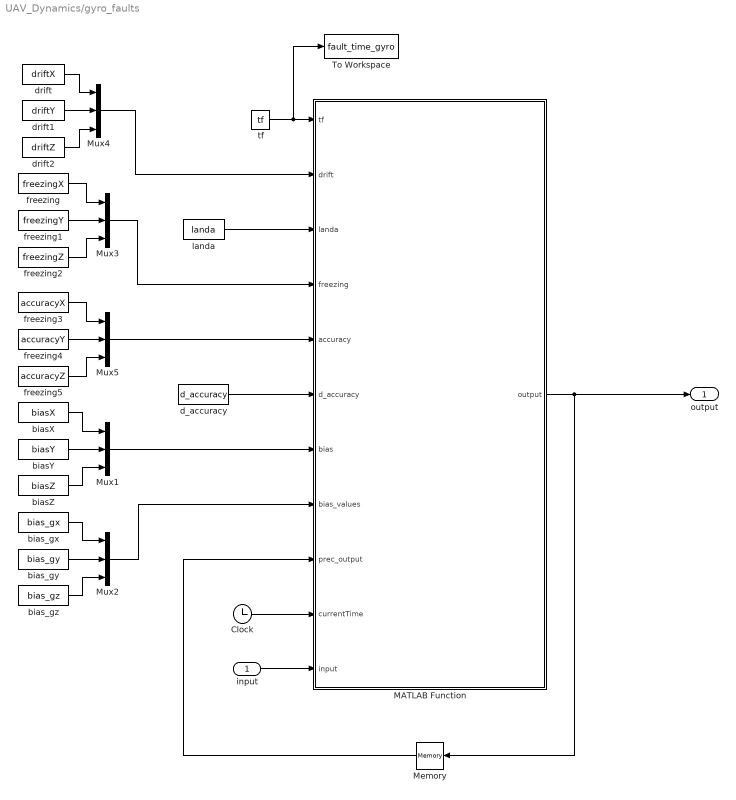
== system UAV_Dynamics/gyro_faults ==
  input : Inport
  Clock : Clock
  MATLAB Function : MATLAB Function  TreatAsAtomicUnit=on
  Memory : Memory
  Mux{1..5} (5 alike) : Mux  Inputs=3
  To Workspace : ToWorkspace  VariableName=fault_time_gyro  SaveFormat=Timeseries  SampleTime=0.01
  biasX : Constant  Value=biasX  SampleTime=0.01
  biasY : Constant  Value=biasY  SampleTime=0.01
  biasZ : Constant  Value=biasZ  SampleTime=0.01
  bias_gx : Constant  Value=bias_gx  SampleTime=0.01
  bias_gy : Constant  Value=bias_gy  SampleTime=0.01
  bias_gz : Constant  Value=bias_gz  SampleTime=0.01
  d_accuracy : Constant  Value=d_accuracy  SampleTime=0.01
  drift : Constant  Value=driftX  SampleTime=0.01
  drift1 : Constant  Value=driftY  SampleTime=0.01
  drift2 : Constant  Value=driftZ  SampleTime=0.01
  freezing : Constant  Value=freezingX  SampleTime=0.01
  freezing1 : Constant  Value=freezingY  SampleTime=0.01
  freezing2 : Constant  Value=freezingZ  SampleTime=0.01
  freezing3 : Constant  Value=accuracyX  SampleTime=0.01
  freezing4 : Constant  Value=accuracyY  SampleTime=0.01
  freezing5 : Constant  Value=accuracyZ  SampleTime=0.01
  landa : Constant  Value=landa  SampleTime=0.01
  tf : Constant  Value=tf
  output : Outport
  wires:
  input/1 -> MATLAB Function/11(input)
  MATLAB Function/1(output) -> output/1, Memory/1
  Memory/1 -> MATLAB Function/9(prec_output)
  d_accuracy/1 -> MATLAB Function/6(d_accuracy)
  Clock/1 -> MATLAB Function/10(currentTime)
  landa/1 -> MATLAB Function/3(landa)
  tf/1 -> To Workspace/1, MATLAB Function/1(tf)
  biasX/1 -> Mux1/1
  biasY/1 -> Mux1/2
  biasZ/1 -> Mux1/3
  bias_gx/1 -> Mux2/1
  bias_gy/1 -> Mux2/2
  bias_gz/1 -> Mux2/3
  Mux1/1 -> MATLAB Function/7(bias)
  Mux2/1 -> MATLAB Function/8(bias_values)
  freezing/1 -> Mux3/1
  freezing1/1 -> Mux3/2
  freezing2/1 -> Mux3/3
  Mux3/1 -> MATLAB Function/4(freezing)
  drift/1 -> Mux4/1
  drift1/1 -> Mux4/2
  drift2/1 -> Mux4/3
  Mux4/1 -> MATLAB Function/2(drift)
  freezing3/1 -> Mux5/1
  freezing4/1 -> Mux5/2
  freezing5/1 -> Mux5/3
  Mux5/1 -> MATLAB Function/5(accuracy)

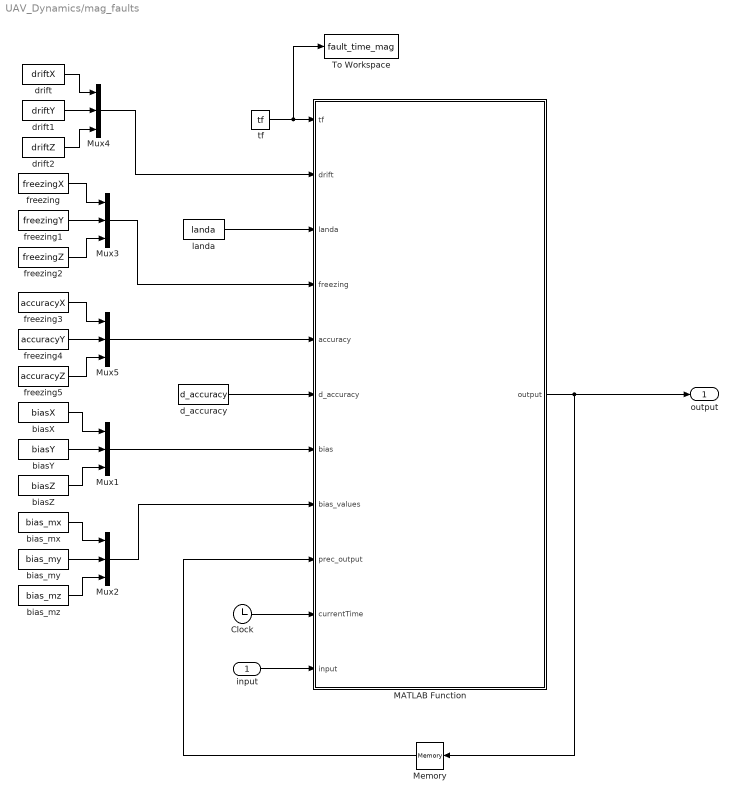
== system UAV_Dynamics/mag_faults ==
  input : Inport
  Clock : Clock
  MATLAB Function : MATLAB Function  TreatAsAtomicUnit=on
  Memory : Memory
  Mux{1..5} (5 alike) : Mux  Inputs=3
  To Workspace : ToWorkspace  VariableName=fault_time_mag  SaveFormat=Timeseries  SampleTime=0.01
  biasX : Constant  Value=biasX  SampleTime=0.01
  biasY : Constant  Value=biasY  SampleTime=0.01
  biasZ : Constant  Value=biasZ  SampleTime=0.01
  bias_mx : Constant  Value=bias_mx  SampleTime=0.01
  bias_my : Constant  Value=bias_my  SampleTime=0.01
  bias_mz : Constant  Value=bias_mz  SampleTime=0.01
  d_accuracy : Constant  Value=d_accuracy  SampleTime=0.01
  drift : Constant  Value=driftX  SampleTime=0.01
  drift1 : Constant  Value=driftY  SampleTime=0.01
  drift2 : Constant  Value=driftZ  SampleTime=0.01
  freezing : Constant  Value=freezingX  SampleTime=0.01
  freezing1 : Constant  Value=freezingY  SampleTime=0.01
  freezing2 : Constant  Value=freezingZ  SampleTime=0.01
  freezing3 : Constant  Value=accuracyX  SampleTime=0.01
  freezing4 : Constant  Value=accuracyY  SampleTime=0.01
  freezing5 : Constant  Value=accuracyZ  SampleTime=0.01
  landa : Constant  Value=landa  SampleTime=0.01
  tf : Constant  Value=tf
  output : Outport
  wires:
  input/1 -> MATLAB Function/11(input)
  MATLAB Function/1(output) -> output/1, Memory/1
  Memory/1 -> MATLAB Function/9(prec_output)
  d_accuracy/1 -> MATLAB Function/6(d_accuracy)
  Clock/1 -> MATLAB Function/10(currentTime)
  landa/1 -> MATLAB Function/3(landa)
  tf/1 -> To Workspace/1, MATLAB Function/1(tf)
  biasX/1 -> Mux1/1
  biasY/1 -> Mux1/2
  biasZ/1 -> Mux1/3
  bias_mx/1 -> Mux2/1
  bias_my/1 -> Mux2/2
  bias_mz/1 -> Mux2/3
  Mux1/1 -> MATLAB Function/7(bias)
  Mux2/1 -> MATLAB Function/8(bias_values)
  freezing/1 -> Mux3/1
  freezing1/1 -> Mux3/2
  freezing2/1 -> Mux3/3
  Mux3/1 -> MATLAB Function/4(freezing)
  drift/1 -> Mux4/1
  drift1/1 -> Mux4/2
  drift2/1 -> Mux4/3
  Mux4/1 -> MATLAB Function/2(drift)
  freezing3/1 -> Mux5/1
  freezing4/1 -> Mux5/2
  freezing5/1 -> Mux5/3
  Mux5/1 -> MATLAB Function/5(accuracy)

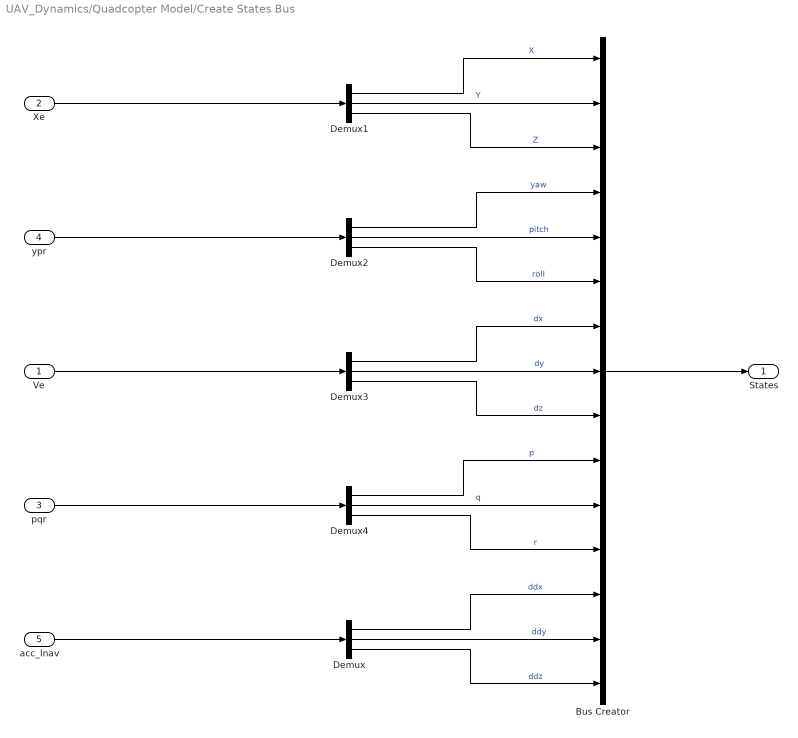
== system UAV_Dynamics/Quadcopter Model/Create States Bus ==
  Ve : Inport
  Xe : Inport  Port=2
  pqr : Inport  Port=3
  ypr : Inport  Port=4
  acc_lnav : Inport  Port=5
  Bus Creator : BusCreator  Inputs=X,Y,Z,yaw,pitch,roll,dx,dy,dz,p,q,r,ddx,ddy,ddz
  Demux{,1..4} (5 alike) : Demux  Outputs=3
  States : Outport
  wires:
  Demux1/1 -> Bus Creator/1  "X"
  Demux1/2 -> Bus Creator/2  "Y"
  ypr/1 -> Demux2/1
  Demux2/2 -> Bus Creator/5  "pitch"
  Demux3/2 -> Bus Creator/8  "dy"
  Demux2/3 -> Bus Creator/6  "roll"
  pqr/1 -> Demux4/1
  Ve/1 -> Demux3/1
  Demux2/1 -> Bus Creator/4  "yaw"
  Demux1/3 -> Bus Creator/3  "Z"
  Demux3/1 -> Bus Creator/7  "dx"
  Demux4/2 -> Bus Creator/11  "q"
  Demux3/3 -> Bus Creator/9  "dz"
  Demux4/3 -> Bus Creator/12  "r"
  Demux4/1 -> Bus Creator/10  "p"
  Bus Creator/1 -> States/1
  Xe/1 -> Demux1/1
  acc_lnav/1 -> Demux/1
  Demux/3 -> Bus Creator/15  "ddz"
  Demux/2 -> Bus Creator/14  "ddy"
  Demux/1 -> Bus Creator/13  "ddx"

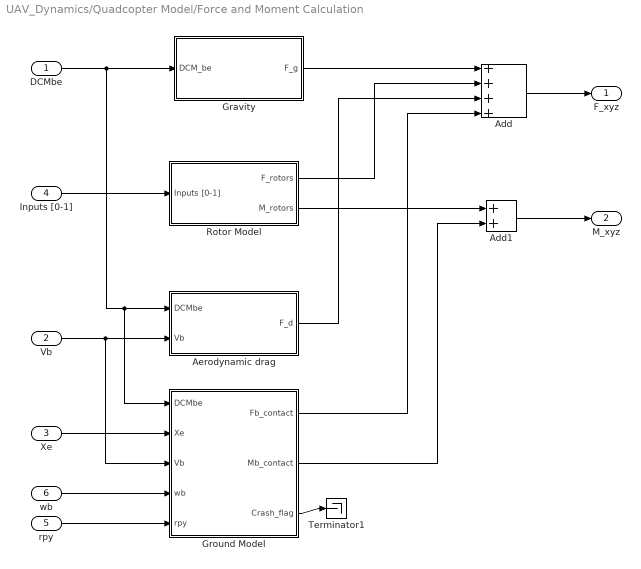
== system UAV_Dynamics/Quadcopter Model/Force and Moment Calculation ==
  DCMbe : Inport
  Vb : Inport  Port=2
  Xe : Inport  Port=3
  Inputs [0-1] : Inport  Port=4
  rpy : Inport  Port=5
  wb : Inport  Port=6
  Add : Sum  Inputs=++++
  Add1 : Sum
  Aerodynamic drag : Subsystem
  Gravity : Subsystem
  Ground Model : Subsystem
  Rotor Model : Subsystem
  Terminator1 : Terminator
  F_xyz : Outport
  M_xyz : Outport  Port=2
  wires:
  Inputs [0-1]/1 -> Rotor Model/1(Inputs [0-1])
  DCMbe/1 -> Ground Model/1(DCMbe), Aerodynamic drag/1(DCMbe), Gravity/1(DCM_be)
  Gravity/1(F_g) -> Add/1
  Add/1 -> F_xyz/1
  Vb/1 -> Ground Model/3(Vb), Aerodynamic drag/2(Vb)
  Rotor Model/1(F_rotors) -> Add/2
  Aerodynamic drag/1(F_d) -> Add/3
  Xe/1 -> Ground Model/2(Xe)
  wb/1 -> Ground Model/4(wb)
  rpy/1 -> Ground Model/5(rpy)
  Rotor Model/2(M_rotors) -> Add1/1
  Ground Model/2(Mb_contact) -> Add1/2
  Add1/1 -> M_xyz/1
  Ground Model/1(Fb_contact) -> Add/4
  Ground Model/3(Crash_flag) -> Terminator1/1

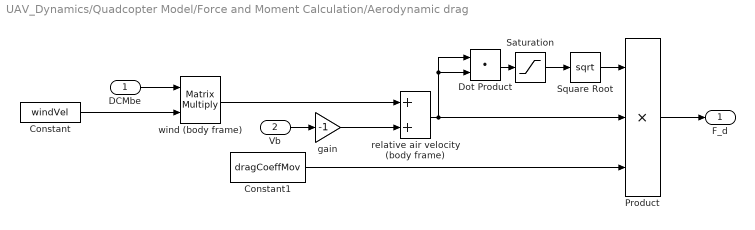
== system UAV_Dynamics/Quadcopter Model/Force and Moment Calculation/Aerodynamic drag ==
  DCMbe : Inport
  Vb : Inport  Port=2
  Constant : Constant  Value=windVel
  Constant1 : Constant  Value=dragCoeffMov
  Dot Product : DotProduct  OutDataTypeStr=Inherit: Inherit via internal rule
  Product : Product  Inputs=3
  Saturation : Saturate  UpperLimit=inf  LowerLimit=0.0001
  Square Root : Sqrt
  gain : Gain  Gain=-1
  relative air velocity (body frame) : Sum
  wind (body frame) : Product  Multiplication=Matrix(*)
  F_d : Outport
  wires:
  relative air velocity (body frame)/1 -> Dot Product/2, Dot Product/1, Product/2
  DCMbe/1 -> wind (body frame)/1
  Product/1 -> F_d/1
  Saturation/1 -> Square Root/1
  Vb/1 -> gain/1
  Dot Product/1 -> Saturation/1
  Square Root/1 -> Product/1
  wind (body frame)/1 -> relative air velocity (body frame)/1
  gain/1 -> relative air velocity (body frame)/2
  Constant1/1 -> Product/3
  Constant/1 -> wind (body frame)/2

== system UAV_Dynamics/Quadcopter Model/Force and Moment Calculation/Gravity ==
  DCM_be : Inport
  Constant : Constant  Value=[0 0 g]'
  Gain : Gain  Gain=mass
  Matrix Multiply : Product  Multiplication=Matrix(*)
  F_g : Outport
  wires:
  Matrix Multiply/1 -> Gain/1
  Constant/1 -> Matrix Multiply/2
  DCM_be/1 -> Matrix Multiply/1
  Gain/1 -> F_g/1

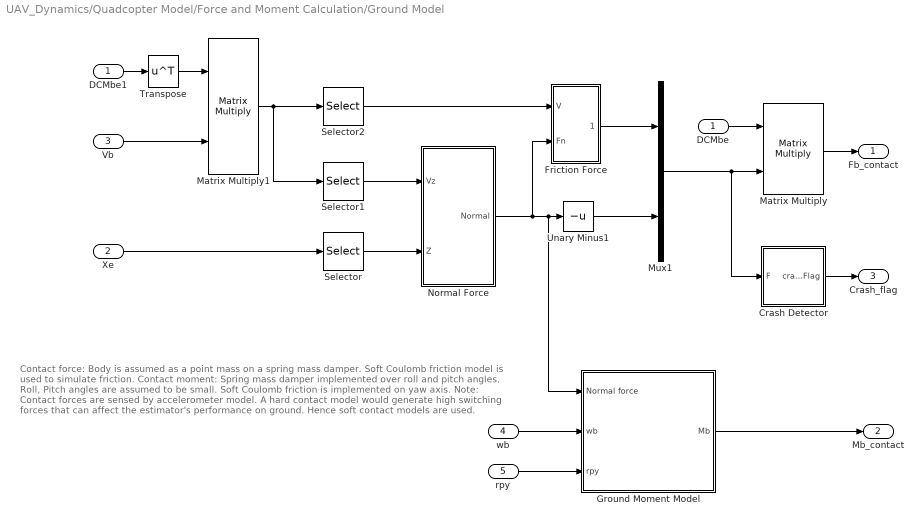
== system UAV_Dynamics/Quadcopter Model/Force and Moment Calculation/Ground Model ==
  note: Contact force:
      | Body is assumed as a point mass on a spring mass damper. Soft Coulomb friction model is used to simulate friction.
      |
      | Contact moment:
      | Spring mass damper implemented over roll and pitch angles. Roll, Pitch angles are assumed to be small.
      | Soft Coulomb friction is implemented on yaw axis.
      |
      | Note:
      | Contact forces are sensed by accelerometer model. A hard contact model would generate high switching forces that can affect the estimator's performance on ground. Hence soft contact models are used.
  DCMbe : Inport
  Xe : Inport  Port=2
  Vb : Inport  Port=3
  wb : Inport  Port=4
  rpy : Inport  Port=5
  Crash Detector : Subsystem
  DCMbe1 : InportShadow
  Friction Force : Subsystem
  Ground Moment Model : Subsystem
  Matrix Multiply : Product  Multiplication=Matrix(*)
  Matrix Multiply1 : Product  Multiplication=Matrix(*)
  Mux1 : Mux  Inputs=2
  Normal Force : Subsystem
  Selector : Selector  InputPortWidth=3  IndexOptions=Index vector (dialog)  Indices=[3]  OutputSizes=1
  Selector1 : Selector  InputPortWidth=3  IndexOptions=Index vector (dialog)  Indices=[3]  OutputSizes=1
  Selector2 : Selector  InputPortWidth=3  IndexOptions=Index vector (dialog)  Indices=[1,2]  OutputSizes=1
  Transpose : Math  Operator=transpose
  Unary Minus1 : UnaryMinus
  Fb_contact : Outport
  Mb_contact : Outport  Port=2
  Crash_flag : Outport  Port=3
  wires:
  Crash Detector/1(crashFlag) -> Crash_flag/1
  Xe/1 -> Selector/1
  Selector1/1 -> Normal Force/1(Vz)
  Selector/1 -> Normal Force/2(Z)
  DCMbe/1 -> Matrix Multiply/1
  Matrix Multiply/1 -> Fb_contact/1
  Normal Force/1(Normal) -> Ground Moment Model/1(Normal force), Unary Minus1/1, Friction Force/2(Fn)
  Mux1/1 -> Crash Detector/1(F), Matrix Multiply/2
  Unary Minus1/1 -> Mux1/2
  Selector2/1 -> Friction Force/1(V)
  Friction Force/1(Friction) -> Mux1/1
  DCMbe1/1 -> Transpose/1
  Transpose/1 -> Matrix Multiply1/1
  Vb/1 -> Matrix Multiply1/2
  Matrix Multiply1/1 -> Selector1/1, Selector2/1
  wb/1 -> Ground Moment Model/2(wb)
  rpy/1 -> Ground Moment Model/3(rpy)
  Ground Moment Model/1(Mb) -> Mb_contact/1

== system UAV_Dynamics/Quadcopter Model/Force and Moment Calculation/Rotor Model ==
  Inputs [0-1] : Inport
  Constant : Constant  Value=rotorPositions
  Constant1 : Constant  Value=rotorDir
  MATLAB Function : MATLAB Function  TreatAsAtomicUnit=on
  Thrust model : Subsystem
  Torque model : Subsystem
  F_rotors : Outport
  M_rotors : Outport  Port=2
  wires:
  Inputs [0-1]/1 -> Torque model/1(In1), Thrust model/1(In1)
  MATLAB Function/1(netF) -> F_rotors/1
  MATLAB Function/2(netM) -> M_rotors/1
  Constant/1 -> MATLAB Function/3(rotorPositions)
  Constant1/1 -> MATLAB Function/4(rotorDir)
  Torque model/1(Out1) -> MATLAB Function/2(tauEachRotor)
  Thrust model/1(Out1) -> MATLAB Function/1(thrustEachRotor)

== system UAV_Dynamics/Quadcopter Model/Force and Moment Calculation/Ground Model/Crash Detector ==
  F : Inport
  Compare To Constant : simulink/Logic and Bit Operations/Compare To Constant  relop=>  const=100  OutDataTypeStr=boolean
  Gain : Gain  Gain=1/mass/g
  norm1 : Subsystem
  crashFlag : Outport
  wires:
  F/1 -> norm1/1(F)
  norm1/1(Out1) -> Gain/1
  Compare To Constant/1 -> crashFlag/1
  Gain/1 -> Compare To Constant/1  "g's"

== system UAV_Dynamics/Quadcopter Model/Force and Moment Calculation/Ground Model/Friction Force ==
  V : Inport
  Fn : Inport  Port=2
  Product : Product
  Saturation : Saturate  UpperLimit=contact.translation.maxFriction  LowerLimit=-contact.translation.maxFriction
  Soft Coulomb Friction : Subsystem
  Unary Minus : UnaryMinus
  Friction : Outport
  wires:
  Fn/1 -> Product/2
  Soft Coulomb Friction/1(Out1) -> Product/1
  Product/1 -> Unary Minus/1
  V/1 -> Soft Coulomb Friction/1(In1)
  Unary Minus/1 -> Saturation/1
  Saturation/1 -> Friction/1

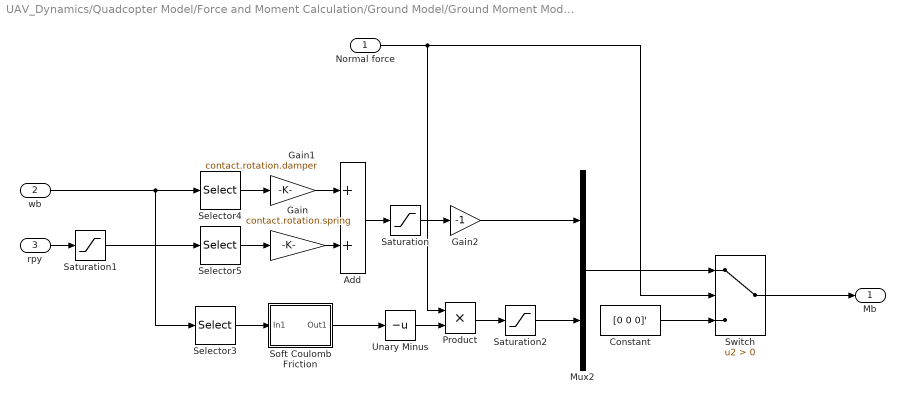
== system UAV_Dynamics/Quadcopter Model/Force and Moment Calculation/Ground Model/Ground Moment Model ==
  Normal force : Inport
  wb : Inport  Port=2
  rpy : Inport  Port=3
  Add : Sum
  Constant : Constant  Value=[0 0 0]'
  Gain : Gain  Gain=contact.rotation.spring
  Gain1 : Gain  Gain=contact.rotation.damper
  Gain2 : Gain  Gain=-1
  Mux2 : Mux  Inputs=2
  Product : Product
  Saturation : Saturate  UpperLimit=control.rotation.maxMoment  LowerLimit=-control.rotation.maxMoment
  Saturation1 : Saturate  UpperLimit=20*pi/180  LowerLimit=-20*pi/180
  Saturation2 : Saturate  UpperLimit=control.rotation.maxMoment  LowerLimit=-control.rotation.maxMoment
  Selector3 : Selector  InputPortWidth=3  IndexOptions=Index vector (dialog)  Indices=[3]  OutputSizes=1
  Selector4 : Selector  InputPortWidth=3  IndexOptions=Index vector (dialog)  Indices=[1, 2]  OutputSizes=1
  Selector5 : Selector  InputPortWidth=3  IndexOptions=Index vector (dialog)  Indices=[1, 2]  OutputSizes=1
  Soft Coulomb Friction : Subsystem
  Switch : Switch  Criteria=u2 > Threshold  SaturateOnIntegerOverflow=off  InputSameDT=off
  Unary Minus : UnaryMinus
  Mb : Outport
  wires:
  Gain2/1 -> Mux2/1
  Add/1 -> Saturation/1
  Gain/1 -> Add/2
  Saturation/1 -> Gain2/1
  Selector4/1 -> Gain1/1
  Gain1/1 -> Add/1
  Constant/1 -> Switch/3
  Selector5/1 -> Gain/1
  Switch/1 -> Mb/1
  Mux2/1 -> Switch/1
  Normal force/1 -> Product/1, Switch/2
  rpy/1 -> Saturation1/1
  Saturation1/1 -> Selector5/1
  wb/1 -> Selector4/1, Selector3/1
  Selector3/1 -> Soft Coulomb Friction/1(In1)
  Soft Coulomb Friction/1(Out1) -> Unary Minus/1
  Unary Minus/1 -> Product/2
  Product/1 -> Saturation2/1
  Saturation2/1 -> Mux2/2

== system UAV_Dynamics/Quadcopter Model/Force and Moment Calculation/Ground Model/Normal Force ==
  Vz : Inport
  Z : Inport  Port=2
  Add : Sum
  Constant : Constant  Value=0
  Damper Kp : Gain  Gain=-contact.translation.damper
  Saturation : Saturate  UpperLimit=contact.translation.maxNormal  LowerLimit=0
  Spring Kp : Gain  Gain=-contact.translation.spring
  Switch : Switch  Criteria=u2 > Threshold  SaturateOnIntegerOverflow=off  InputSameDT=off
  Unary Minus : UnaryMinus
  Unary Minus1 : UnaryMinus
  Normal : Outport
  wires:
  Constant/1 -> Switch/1
  Z/1 -> Unary Minus/1
  Switch/1 -> Saturation/1
  Damper Kp/1 -> Add/2
  Add/1 -> Switch/3
  Spring Kp/1 -> Add/1
  Vz/1 -> Unary Minus1/1
  Saturation/1 -> Normal/1
  Unary Minus/1 -> Spring Kp/1, Switch/2
  Unary Minus1/1 -> Damper Kp/1

== system UAV_Dynamics/Quadcopter Model/Force and Moment Calculation/Rotor Model/Thrust model ==
  In1 : Inport
  Demux : Demux
  Mux : Mux
  Transfer Fcn{,2..4} (4 alike) : TransferFcn  Numerator=[rotorThrustMax]  Denominator=[rotorTimeConst 1]
  Out1 : Outport
  wires:
  Transfer Fcn3/1 -> Mux/2
  Demux/1 -> Transfer Fcn4/1
  Transfer Fcn2/1 -> Mux/3
  Demux/3 -> Transfer Fcn2/1
  Mux/1 -> Out1/1
  Transfer Fcn4/1 -> Mux/1
  Demux/4 -> Transfer Fcn/1
  Demux/2 -> Transfer Fcn3/1
  Transfer Fcn/1 -> Mux/4
  In1/1 -> Demux/1

== system UAV_Dynamics/Quadcopter Model/Force and Moment Calculation/Rotor Model/Torque model ==
  In1 : Inport
  Demux : Demux
  Mux : Mux
  Transfer Fcn{1..4} (4 alike) : TransferFcn  Numerator=[rotorTorqueMax]  Denominator=[rotorTimeConst 1]
  Out1 : Outport
  wires:
  Transfer Fcn4/1 -> Mux/4
  Demux/1 -> Transfer Fcn1/1
  Transfer Fcn3/1 -> Mux/3
  Transfer Fcn2/1 -> Mux/2
  Demux/2 -> Transfer Fcn2/1
  Demux/4 -> Transfer Fcn4/1
  Demux/3 -> Transfer Fcn3/1
  Mux/1 -> Out1/1
  Transfer Fcn1/1 -> Mux/1
  In1/1 -> Demux/1

== system UAV_Dynamics/Quadcopter Model/Force and Moment Calculation/Ground Model/Crash Detector/norm1 ==
  F : Inport
  Dot Product : DotProduct  OutDataTypeStr=Inherit: Inherit via internal rule
  Sqrt : Sqrt
  Out1 : Outport
  wires:
  Dot Product/1 -> Sqrt/1
  F/1 -> Dot Product/2, Dot Product/1
  Sqrt/1 -> Out1/1

== system UAV_Dynamics/Quadcopter Model/Force and Moment Calculation/Ground Model/Friction Force/Soft Coulomb Friction ==
  note: Pennestrì, E., Rossi, V., Salvini, P. et al. Review and comparison of dry friction force models. Nonlinear Dyn 83, 1785–1801 (2016). https://doi.org/10.1007/s11071-015-2485-3
  In1 : Inport
  Tanh : Trigonometry  Operator=tanh
  friction coefficient : Gain  Gain=contact.translation.friction
  vd : Gain  Gain=1/contact.translation.vd
  Out1 : Outport
  wires:
  In1/1 -> vd/1
  vd/1 -> Tanh/1
  Tanh/1 -> friction coefficient/1
  friction coefficient/1 -> Out1/1

== system UAV_Dynamics/Quadcopter Model/Force and Moment Calculation/Ground Model/Ground Moment Model/Soft Coulomb Friction ==
  note: Pennestrì, E., Rossi, V., Salvini, P. et al. Review and comparison of dry friction force models. Nonlinear Dyn 83, 1785–1801 (2016). https://doi.org/10.1007/s11071-015-2485-3
  In1 : Inport
  Tanh : Trigonometry  Operator=tanh
  friction coefficient : Gain  Gain=control.rotation.friction
  vd : Gain  Gain=1/control.rotation.vd
  Out1 : Outport
  wires:
  In1/1 -> vd/1
  vd/1 -> Tanh/1
  Tanh/1 -> friction coefficient/1
  friction coefficient/1 -> Out1/1

== matlab function UAV_Dynamics/gps_faults/MATLAB Function ==
  settings: updateMethod=DISCRETE
  data: tf input; gps_accuracy input; loss_signal input; lossProbability input; currentTime input; input input; output output; accuracyErrorMeters input

function output  = GPS_fault(tf, gps_accuracy, loss_signal, lossProbability, ...
    currentTime, input, accuracyErrorMeters)
        
    output = input;
   
    if (currentTime >= tf )
        % Packet Loss Simulation
        if(loss_signal)
            lossProbability = lossProbability/100;
            % rand returns a random scalar drawn from the uniform distribution in the interval (0,1)
            if rand < lossProbability
                output = zeros(size(input)); 
            end
        end

        if(gps_accuracy)
            meters_per_degree_lat = 111320;  % Latitude approximation
            meters_per_degree_lon = meters_per_degree_lat * cosd(output(2));  
            
            % Genereting random error
            error_lat = randn(1) * (accuracyErrorMeters / meters_per_degree_lat);
            error_lon = randn(1) * (accuracyErrorMeters / meters_per_degree_lon);
            
            % Add error to coordinates
            output(1) = input(1) + error_lat;
            output(2) = input(2) + error_lon;
        end  
    
    end

end

== matlab function UAV_Dynamics/Buffer1/MATLAB Function ==
  data: buffer input; buffer output; newValue input; bufferSize input; k input; k output
function [buffer, k] = writeCircularBuffer(buffer, newValue, bufferSize, k)

    % Funzione per implementare un buffer circolare con indice
    % buffer: il buffer corrente (array)
    % newValue: il nuovo valore da aggiungere
    % bufferSize: la dimensione massima del buffer
    % k: indice dell'inizio del buffer circolar
 
    % Inserisci il nuovo valore nella posizione corretta
    buffer(k) = newValue;
 
    % Aggiorna l'indice k per il prossimo elemento
    k = mod(k, bufferSize) + 1;
end
